simulink model "hebing"  (R2016b)
settings: Solver=VariableStepAuto  StartTime=0.0  StopTime=10000  RelTol=1e-3
libraries: simulink x4
settings Model: Creator=黄天  LastModifiedBy=XuanjieXiao

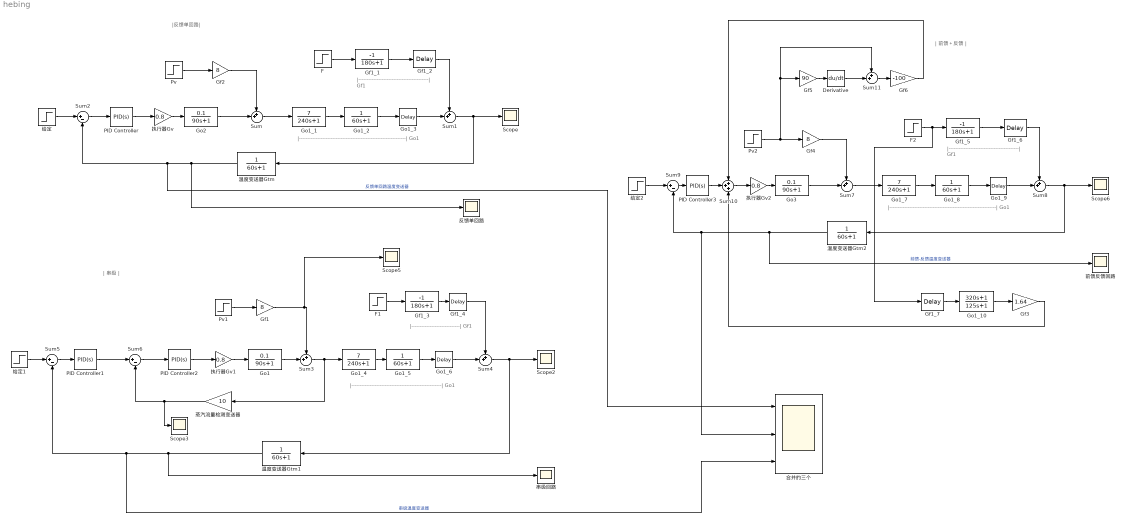
== system hebing ==
  note: |----------------------------------------------------------------|
      | Go1
  note: |------------------------------------------|
      | Gf1
  note: |------------------------------------------------------|
      | Go1
  note: |-----------------------------|
      | Gf1
  note: |----------------------------------------------------------------|
      | Go1
  note: |------------------------------------------|
      | Gf1
  note: |反馈单回路|
  note: | 串级 |
  note: | 前馈＋反馈 |
  Derivative : Derivative
  F : Step  Time=7500  After=0  SampleTime=0
  F1 : Step  Time=7500  After=0  SampleTime=0
  F2 : Step  Time=7500  After=0  SampleTime=0
  Gf1 : Gain  Gain=8
  Gf1_1 : TransferFcn  Numerator=[-1]  Denominator=[180 1]
  Gf1_2 : TransportDelay  DelayTime=180
  Gf1_3 : TransferFcn  Numerator=[-1]  Denominator=[180 1]
  Gf1_4 : TransportDelay  DelayTime=180
  Gf1_5 : TransferFcn  Numerator=[-1]  Denominator=[180 1]
  Gf1_6 : TransportDelay  DelayTime=180
  Gf1_7 : TransportDelay  DelayTime=40
  Gf2 : Gain  Gain=8
  Gf3 : Gain  Gain=1.64
  Gf4 : Gain  Gain=8
  Gf5 : Gain  Gain=90
  Gf6 : Gain  Gain=-100
  Go1 : TransferFcn  Numerator=[0.1]  Denominator=[90 1]
  Go1_1 : TransferFcn  Numerator=[7]  Denominator=[240 1]
  Go1_10 : TransferFcn  Numerator=[320 1]  Denominator=[125 1]
  Go1_2 : TransferFcn  Denominator=[60 1]
  Go1_3 : TransportDelay  DelayTime=60
  Go1_4 : TransferFcn  Numerator=[7]  Denominator=[240 1]
  Go1_5 : TransferFcn  Denominator=[60 1]
  Go1_6 : TransportDelay  DelayTime=60
  Go1_7 : TransferFcn  Numerator=[7]  Denominator=[240 1]
  Go1_8 : TransferFcn  Denominator=[60 1]
  Go1_9 : TransportDelay  DelayTime=60
  Go2 : TransferFcn  Numerator=[0.1]  Denominator=[90 1]
  Go3 : TransferFcn  Numerator=[0.1]  Denominator=[90 1]
  PID Controller : simulink/Continuous/PID Controller  Controller=PID  TimeDomain=Continuous-time  SampleTime=-1  IntegratorMethod=Forward Euler  FilterMethod=Forward Euler  Form=Parallel  UseFilter=on  ControllerParametersSource=internal  P=0.83  I=0.00255  D=0  N=1  InitialConditionSource=internal  InitialConditionForIntegrator=0  InitialConditionForFilter=0  ExternalReset=none  LimitOutput=off  UpperSaturationLimit=inf  LowerSaturationLimit=-inf  LinearizeAsGain=on  AntiWindupMode=none  Kb=1  TrackingMode=off  Kt=1  PParamMin=[]  PParamMax=[]  IParamMin=[]  IParamMax=[]  DParamMin=[]  DParamMax=[]  NParamMin=[]  NParamMax=[]  KbParamMin=[]  KbParamMax=[]  KtParamMin=[]  KtParamMax=[]  POutMin=[]  POutMax=[]  IOutMin=[]  IOutMax=[]  DOutMin=[]  DOutMax=[]  NOutMin=[]  NOutMax=[]  KbOutMin=[]  KbOutMax=[]  KtOutMin=[]  KtOutMax=[]  IntegratorOutMin=[]  IntegratorOutMax=[]  FilterOutMin=[]  FilterOutMax=[]  SumOutMin=[]  SumOutMax=[]  SumI1OutMin=[]  SumI1OutMax=[]  SumI2OutMin=[]  SumI2OutMax=[]  SumI3OutMin=[]  SumI3OutMax=[]  SumDOutMin=[]  SumDOutMax=[]  SaturationOutMin=[]  SaturationOutMax=[]  IntegratorContinuousStateAttributes=''  IntegratorStateMustResolveToSignalObject=off  IntegratorRTWStateStorageClass=Auto  FilterContinuousStateAttributes=''  FilterStateMustResolveToSignalObject=off  FilterRTWStateStorageClass=Auto  DifferentiatorICPrevScaledInput=0  DifferentiatorOutMin=[]  DifferentiatorOutMax=[]
  PID Controller1 : simulink/Continuous/PID Controller  Controller=PID  TimeDomain=Continuous-time  SampleTime=-1  IntegratorMethod=Forward Euler  FilterMethod=Forward Euler  Form=Parallel  UseFilter=on  ControllerParametersSource=internal  P=2.92  I=0.0075  D=251.97462  N=1  InitialConditionSource=internal  InitialConditionForIntegrator=0  InitialConditionForFilter=0  ExternalReset=none  LimitOutput=off  UpperSaturationLimit=inf  LowerSaturationLimit=-inf  LinearizeAsGain=on  AntiWindupMode=none  Kb=1  TrackingMode=off  Kt=1  PParamMin=[]  PParamMax=[]  IParamMin=[]  IParamMax=[]  DParamMin=[]  DParamMax=[]  NParamMin=[]  NParamMax=[]  KbParamMin=[]  KbParamMax=[]  KtParamMin=[]  KtParamMax=[]  POutMin=[]  POutMax=[]  IOutMin=[]  IOutMax=[]  DOutMin=[]  DOutMax=[]  NOutMin=[]  NOutMax=[]  KbOutMin=[]  KbOutMax=[]  KtOutMin=[]  KtOutMax=[]  IntegratorOutMin=[]  IntegratorOutMax=[]  FilterOutMin=[]  FilterOutMax=[]  SumOutMin=[]  SumOutMax=[]  SumI1OutMin=[]  SumI1OutMax=[]  SumI2OutMin=[]  SumI2OutMax=[]  SumI3OutMin=[]  SumI3OutMax=[]  SumDOutMin=[]  SumDOutMax=[]  SaturationOutMin=[]  SaturationOutMax=[]  IntegratorContinuousStateAttributes=''  IntegratorStateMustResolveToSignalObject=off  IntegratorRTWStateStorageClass=Auto  FilterContinuousStateAttributes=''  FilterStateMustResolveToSignalObject=off  FilterRTWStateStorageClass=Auto  DifferentiatorICPrevScaledInput=0  DifferentiatorOutMin=[]  DifferentiatorOutMax=[]
  PID Controller2 : simulink/Continuous/PID Controller  Controller=PID  TimeDomain=Continuous-time  SampleTime=-1  IntegratorMethod=Forward Euler  FilterMethod=Forward Euler  Form=Parallel  UseFilter=on  ControllerParametersSource=internal  P=9  I=0.235  D=0  N=1  InitialConditionSource=internal  InitialConditionForIntegrator=0  InitialConditionForFilter=0  ExternalReset=none  LimitOutput=off  UpperSaturationLimit=inf  LowerSaturationLimit=-inf  LinearizeAsGain=on  AntiWindupMode=none  Kb=1  TrackingMode=off  Kt=1  PParamMin=[]  PParamMax=[]  IParamMin=[]  IParamMax=[]  DParamMin=[]  DParamMax=[]  NParamMin=[]  NParamMax=[]  KbParamMin=[]  KbParamMax=[]  KtParamMin=[]  KtParamMax=[]  POutMin=[]  POutMax=[]  IOutMin=[]  IOutMax=[]  DOutMin=[]  DOutMax=[]  NOutMin=[]  NOutMax=[]  KbOutMin=[]  KbOutMax=[]  KtOutMin=[]  KtOutMax=[]  IntegratorOutMin=[]  IntegratorOutMax=[]  FilterOutMin=[]  FilterOutMax=[]  SumOutMin=[]  SumOutMax=[]  SumI1OutMin=[]  SumI1OutMax=[]  SumI2OutMin=[]  SumI2OutMax=[]  SumI3OutMin=[]  SumI3OutMax=[]  SumDOutMin=[]  SumDOutMax=[]  SaturationOutMin=[]  SaturationOutMax=[]  IntegratorContinuousStateAttributes=''  IntegratorStateMustResolveToSignalObject=off  IntegratorRTWStateStorageClass=Auto  FilterContinuousStateAttributes=''  FilterStateMustResolveToSignalObject=off  FilterRTWStateStorageClass=Auto  DifferentiatorICPrevScaledInput=0  DifferentiatorOutMin=[]  DifferentiatorOutMax=[]
  PID Controller3 : simulink/Continuous/PID Controller  Controller=PID  TimeDomain=Continuous-time  SampleTime=-1  IntegratorMethod=Forward Euler  FilterMethod=Forward Euler  Form=Parallel  UseFilter=on  ControllerParametersSource=internal  P=0.83  I=0.00255  D=0  N=1  InitialConditionSource=internal  InitialConditionForIntegrator=0  InitialConditionForFilter=0  ExternalReset=none  LimitOutput=off  UpperSaturationLimit=inf  LowerSaturationLimit=-inf  LinearizeAsGain=on  AntiWindupMode=none  Kb=1  TrackingMode=off  Kt=1  PParamMin=[]  PParamMax=[]  IParamMin=[]  IParamMax=[]  DParamMin=[]  DParamMax=[]  NParamMin=[]  NParamMax=[]  KbParamMin=[]  KbParamMax=[]  KtParamMin=[]  KtParamMax=[]  POutMin=[]  POutMax=[]  IOutMin=[]  IOutMax=[]  DOutMin=[]  DOutMax=[]  NOutMin=[]  NOutMax=[]  KbOutMin=[]  KbOutMax=[]  KtOutMin=[]  KtOutMax=[]  IntegratorOutMin=[]  IntegratorOutMax=[]  FilterOutMin=[]  FilterOutMax=[]  SumOutMin=[]  SumOutMax=[]  SumI1OutMin=[]  SumI1OutMax=[]  SumI2OutMin=[]  SumI2OutMax=[]  SumI3OutMin=[]  SumI3OutMax=[]  SumDOutMin=[]  SumDOutMax=[]  SaturationOutMin=[]  SaturationOutMax=[]  IntegratorContinuousStateAttributes=''  IntegratorStateMustResolveToSignalObject=off  IntegratorRTWStateStorageClass=Auto  FilterContinuousStateAttributes=''  FilterStateMustResolveToSignalObject=off  FilterRTWStateStorageClass=Auto  DifferentiatorICPrevScaledInput=0  DifferentiatorOutMin=[]  DifferentiatorOutMax=[]
  Pv : Step  Time=3000  After=0  SampleTime=0
  Pv1 : Step  Time=3000  After=0  SampleTime=0
  Pv2 : Step  Time=3000  After=0  SampleTime=0
  Scope{,2..3,5..6} (5 alike) : Scope
  Sum{,1,3..4,7..8,11} (7 alike) : Sum  Inputs=++|
  Sum10 : Sum  Inputs=+++
  Sum{2,5..6,9} (4 alike) : Sum  Inputs=|+-
  串级回路 : Scope
  前馈反馈回路 : Scope
  反馈单回路 : Scope
  合并的三个 : Scope  NumInputPorts=3
  执行器Gv : Gain  Gain=0.8
  执行器Gv1 : Gain  Gain=0.8
  执行器Gv2 : Gain  Gain=0.8
  温度变送器Gtm : TransferFcn  Denominator=[60 1]
  温度变送器Gtm1 : TransferFcn  Denominator=[60 1]
  温度变送器Gtm2 : TransferFcn  Denominator=[60 1]
  给定 : Step  After=10  SampleTime=0
  给定1 : Step  Time=0  After=10  SampleTime=0
  给定2 : Step  After=10  SampleTime=0
  蒸汽流量检测变送器 : Gain  Gain=10
  wires:
  Go1_2/1 -> Go1_3/1
  Go1_1/1 -> Go1_2/1
  Gf1_1/1 -> Gf1_2/1
  Go1_3/1 -> Sum1/2
  Sum/1 -> Go1_1/1
  Sum1/1 -> 温度变送器Gtm/1, Scope/1
  温度变送器Gtm/1 -> 反馈单回路/1, 合并的三个/1, Sum2/2  "反馈单回路温度变送器"
  给定/1 -> Sum2/1
  Go2/1 -> Sum/2
  执行器Gv/1 -> Go2/1
  Sum2/1 -> PID Controller/1
  PID Controller/1 -> 执行器Gv/1
  F/1 -> Gf1_1/1
  Gf1_2/1 -> Sum1/1
  Pv/1 -> Gf2/1
  Gf2/1 -> Sum/1
  Go1_5/1 -> Go1_6/1
  Go1_4/1 -> Go1_5/1
  Gf1_3/1 -> Gf1_4/1
  Go1_6/1 -> Sum4/2
  Sum3/1 -> Go1_4/1, 蒸汽流量检测变送器/1
  Sum4/1 -> 温度变送器Gtm1/1, Scope2/1
  温度变送器Gtm1/1 -> 串级回路/1, 合并的三个/3, Sum5/2  "串级温度变送器"
  给定1/1 -> Sum5/1
  Go1/1 -> Sum3/2
  Sum6/1 -> PID Controller2/1
  蒸汽流量检测变送器/1 -> Scope3/1, Sum6/2
  执行器Gv1/1 -> Go1/1
  PID Controller2/1 -> 执行器Gv1/1
  Sum5/1 -> PID Controller1/1
  Gf1/1 -> Scope5/1, Sum3/1
  F1/1 -> Gf1_3/1
  Gf1_4/1 -> Sum4/1
  Pv1/1 -> Gf1/1
  PID Controller1/1 -> Sum6/1
  Go1_8/1 -> Go1_9/1
  Go1_7/1 -> Go1_8/1
  Gf1_5/1 -> Gf1_6/1
  Go1_9/1 -> Sum8/2
  Sum7/1 -> Go1_7/1
  Sum8/1 -> 温度变送器Gtm2/1, Scope6/1
  温度变送器Gtm2/1 -> 前馈反馈回路/1, Sum9/2, 合并的三个/2  "前馈-反馈温度变送器"
  给定2/1 -> Sum9/1
  Go3/1 -> Sum7/2
  执行器Gv2/1 -> Go3/1
  Sum9/1 -> PID Controller3/1
  F2/1 -> Gf1_7/1, Gf1_5/1
  Gf1_6/1 -> Sum8/1
  Pv2/1 -> Sum11/1, Gf5/1, Gf4/1
  Gf4/1 -> Sum7/1
  Sum10/1 -> 执行器Gv2/1
  Gf1_7/1 -> Go1_10/1
  Go1_10/1 -> Gf3/1
  Gf3/1 -> Sum10/3
  PID Controller3/1 -> Sum10/2
  Gf5/1 -> Derivative/1
  Derivative/1 -> Sum11/2
  Sum11/1 -> Gf6/1
  Gf6/1 -> Sum10/1
